simulink model "net_model_2_nodes_ext_switch"  (R2024a)
settings: Solver=VariableStepAuto  StartTime=0.0  StopTime=n_max  RelTol=1e-3
values from neighbouring files (symbols this model uses):
  node_1_0 = [0; 0]    [compute_controller.m]    (also in main.m = [5; 1])
  node_2_0 = [0; 0]    [compute_controller.m]    (also in main.m = [1; 1])
  ss_ctr_fault = ss(ss_fault.A + L2 * ss_fault.C + ss_fault.B * J2, -L2, J2, 0, 1)    [compute_controller.m]
  ss_ctr_nom = ss(ss_nom.A + L1 * ss_nom.C + ss_nom.B * J1, -L1, J1, 0, 1)    [compute_controller.m]
  ss_fault = ss(A, B, C, 0, 1)    [compute_controller.m]
  ss_nom = ss(A, B, C, 0, 1)    [compute_controller.m]
settings Model: Creator=antoniostavarache  LastModifiedBy=antoniostavarache

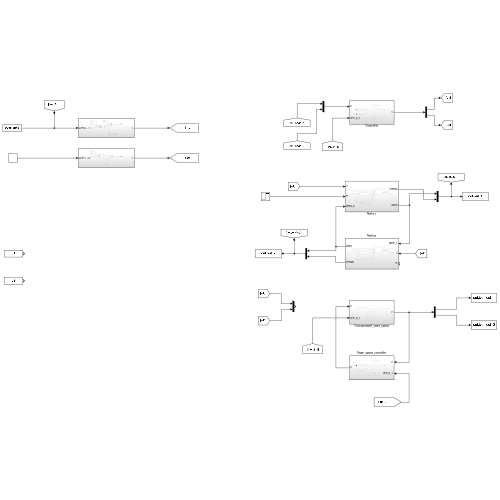
[thumbnail: Simulink's stored preview of the top-level diagram]
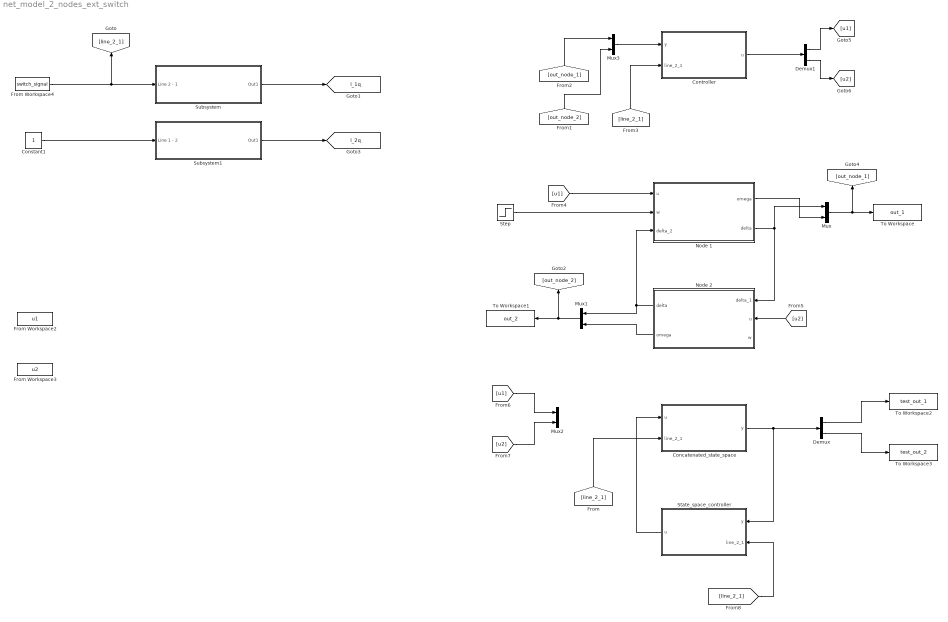
== system net_model_2_nodes_ext_switch ==
  Concatenated_state_space : Subsystem
  Constant1 : Constant
  Controller : Subsystem
  Demux : Demux  Outputs=2
  Demux1 : Demux  Outputs=2
  From Workspace2 : FromWorkspace  VariableName=u1
  From Workspace3 : FromWorkspace  VariableName=u2
  From Workspace4 : FromWorkspace  VariableName=switch_signal  SampleTime=1
  Mux{,1..3} (4 alike) : Mux  Inputs=2
  Node 1 : Subsystem
  Node 2 : Subsystem
  State_space_controller : Subsystem
  Step : Step  Time=250  SampleTime=0
  Subsystem : Subsystem
  Subsystem1 : Subsystem
  To Workspace : ToWorkspace  VariableName=out_1  SaveFormat=Timeseries  SampleTime=-1
  To Workspace1 : ToWorkspace  VariableName=out_2  SaveFormat=Timeseries  SampleTime=-1
  To Workspace2 : ToWorkspace  VariableName=test_out_1  SaveFormat=Timeseries  SampleTime=-1
  To Workspace3 : ToWorkspace  VariableName=test_out_2  SaveFormat=Timeseries  SampleTime=-1
  tag scope: l_1q=global, l_2q=global
  wires:
  Node 1/2(delta) -> Node 2/1(delta_1), Mux/1
  Node 2/1(delta) -> Mux1/1, Node 1/3(delta_2)
  Mux/1 -> To Workspace/1, [out_node_1]
  Mux1/1 -> To Workspace1/1, [out_node_2]
  Node 2/2(omega) -> Mux1/2
  Demux/1 -> To Workspace2/1
  Demux/2 -> To Workspace3/1
  Node 1/1(omega) -> Mux/2
  Subsystem/1(Out1) -> [l_1q]
  Constant1/1 -> Subsystem1/1(Line 1 - 2)
  Subsystem1/1(Out1) -> [l_2q]
  Concatenated_state_space/1(y) -> State_space_controller/1(y), Demux/1
  From Workspace4/1 -> Subsystem/1(Line 2 - 1), [line_2_1]
  [out_node_1] -> Mux3/1
  [out_node_2] -> Mux3/2
  Mux3/1 -> Controller/1(y)
  [line_2_1] -> Controller/2(line_2_1)
  Demux1/1 -> [u1]
  Demux1/2 -> [u2]
  [u1] -> Node 1/1(u)
  [u2] -> Node 2/2(u)
  [line_2_1] -> Concatenated_state_space/2(line_2_1)
  Controller/1(u) -> Demux1/1
  [u1] -> Mux2/1
  [u2] -> Mux2/2
  [line_2_1] -> State_space_controller/2(line_2_1)
  State_space_controller/1(u) -> Concatenated_state_space/1(u)
  Step/1 -> Node 1/2(w)

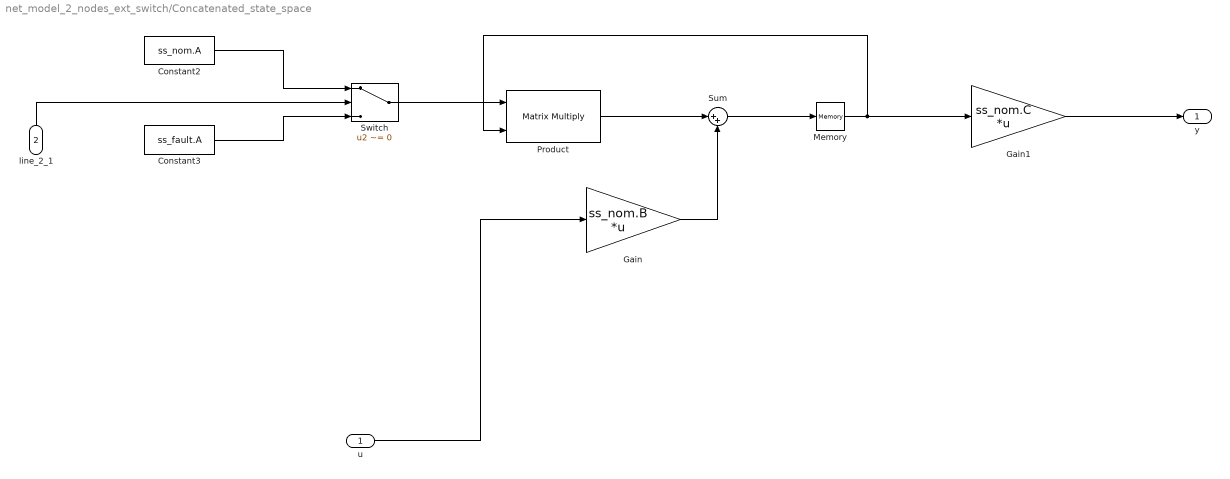
== system net_model_2_nodes_ext_switch/Concatenated_state_space ==
  u : Inport
  line_2_1 : Inport  Port=2
  Constant2 : Constant  Value=ss_nom.A
  Constant3 : Constant  Value=ss_fault.A
  Gain : Gain  Gain=ss_nom.B  Multiplication=Matrix(K*u) (u vector)
  Gain1 : Gain  Gain=ss_nom.C  Multiplication=Matrix(K*u) (u vector)
  Memory : Memory  InitialCondition=[node_1_0; node_2_0]
  Product : Product  Multiplication=Matrix(*)
  Sum : Sum  Inputs=|++
  Switch : Switch  Criteria=u2 ~= 0  SaturateOnIntegerOverflow=off  InputSameDT=off
  y : Outport
  wires:
  Constant3/1 -> Switch/3
  Switch/1 -> Product/1
  Product/1 -> Sum/1
  Memory/1 -> Gain1/1, Product/2
  Gain1/1 -> y/1
  u/1 -> Gain/1
  Sum/1 -> Memory/1
  Gain/1 -> Sum/2
  line_2_1/1 -> Switch/2
  Constant2/1 -> Switch/1

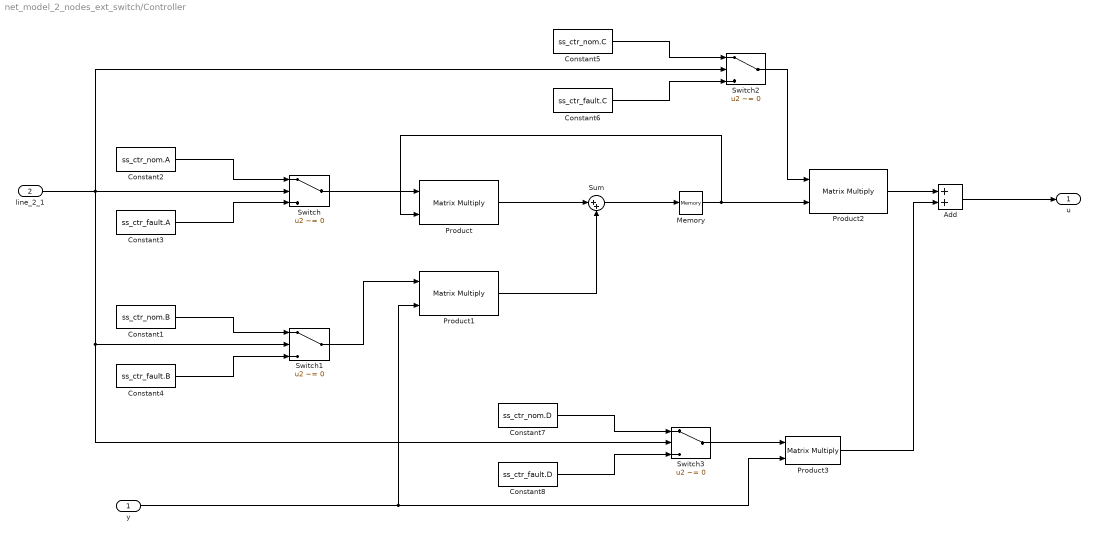
== system net_model_2_nodes_ext_switch/Controller ==
  y : Inport
  line_2_1 : Inport  Port=2
  Add : Sum
  Constant1 : Constant  Value=ss_ctr_nom.B
  Constant2 : Constant  Value=ss_ctr_nom.A
  Constant3 : Constant  Value=ss_ctr_fault.A
  Constant4 : Constant  Value=ss_ctr_fault.B
  Constant5 : Constant  Value=ss_ctr_nom.C
  Constant6 : Constant  Value=ss_ctr_fault.C
  Constant7 : Constant  Value=ss_ctr_nom.D
  Constant8 : Constant  Value=ss_ctr_fault.D
  Memory : Memory  InitialCondition=zeros(4, 1)
  Product{,1..3} (4 alike) : Product  Multiplication=Matrix(*)
  Sum : Sum  Inputs=|++
  Switch{,1..3} (4 alike) : Switch  Criteria=u2 ~= 0  SaturateOnIntegerOverflow=off  InputSameDT=off
  u : Outport
  wires:
  Constant3/1 -> Switch/3
  Switch/1 -> Product/1
  Product/1 -> Sum/1
  Memory/1 -> Product2/2, Product/2
  y/1 -> Product1/2, Product3/2
  Sum/1 -> Memory/1
  Product1/1 -> Sum/2
  line_2_1/1 -> Switch2/2, Switch3/2, Switch1/2, Switch/2
  Constant2/1 -> Switch/1
  Constant4/1 -> Switch1/3
  Constant1/1 -> Switch1/1
  Switch1/1 -> Product1/1
  Constant6/1 -> Switch2/3
  Constant5/1 -> Switch2/1
  Switch2/1 -> Product2/1
  Constant8/1 -> Switch3/3
  Constant7/1 -> Switch3/1
  Product2/1 -> Add/1
  Add/1 -> u/1
  Switch3/1 -> Product3/1
  Product3/1 -> Add/2

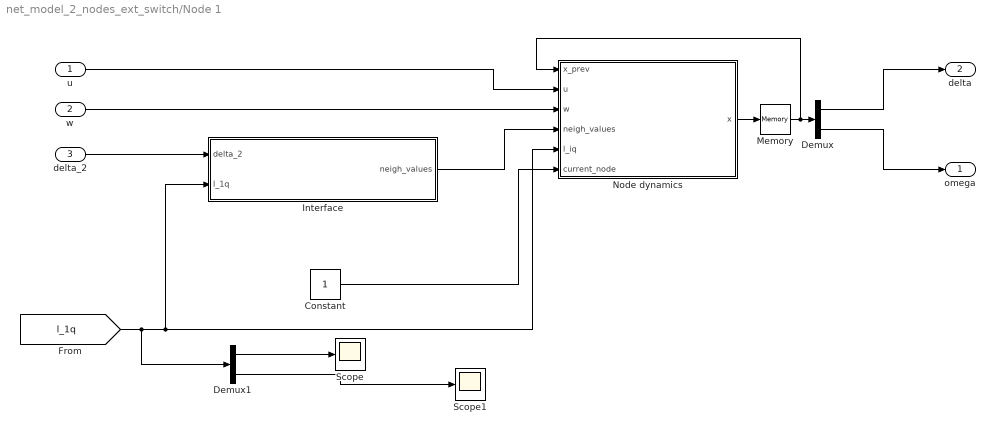
== system net_model_2_nodes_ext_switch/Node 1 ==
  u : Inport
  w : Inport  Port=2
  delta_2 : Inport  Port=3
  Constant : Constant
  Demux : Demux  Outputs=2
  Demux1 : Demux  Outputs=2
  Interface : MATLAB Function  TreatAsAtomicUnit=on
  Memory : Memory  InitialCondition=node_1_0
  Node dynamics : MATLAB Function  TreatAsAtomicUnit=on
  Scope : Scope
  Scope1 : Scope
  omega : Outport
  delta : Outport  Port=2
  wires:
  Node dynamics/1(x) -> Memory/1
  Interface/1(neigh_values) -> Node dynamics/4(neigh_values)
  u/1 -> Node dynamics/2(u)
  w/1 -> Node dynamics/3(w)
  Demux/1 -> delta/1
  Demux/2 -> omega/1
  Memory/1 -> Node dynamics/1(x_prev), Demux/1
  delta_2/1 -> Interface/1(delta_2)
  [l_1q] -> Demux1/1, Node dynamics/5(l_iq), Interface/2(l_1q)
  Constant/1 -> Node dynamics/6(current_node)
  Demux1/1 -> Scope/1
  Demux1/2 -> Scope1/1

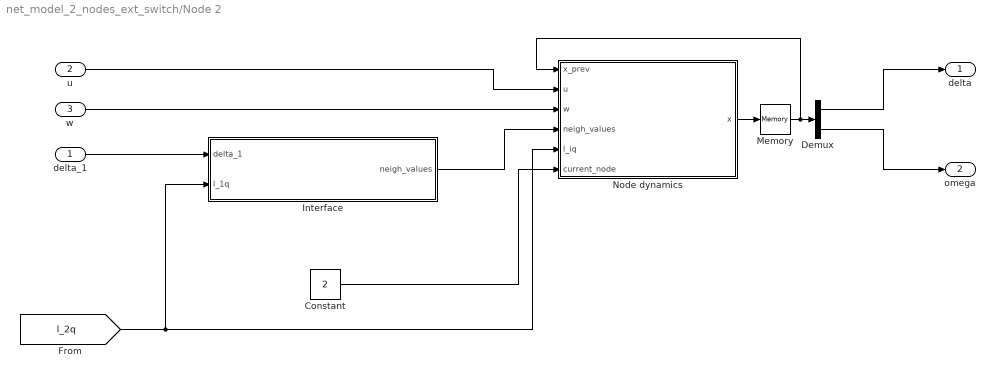
== system net_model_2_nodes_ext_switch/Node 2 ==
  delta_1 : Inport
  u : Inport  Port=2
  w : Inport  Port=3
  Constant : Constant  Value=2
  Demux : Demux  Outputs=2
  Interface : MATLAB Function  TreatAsAtomicUnit=on
  Memory : Memory  InitialCondition=node_2_0
  Node dynamics : MATLAB Function  TreatAsAtomicUnit=on
  delta : Outport
  omega : Outport  Port=2
  wires:
  Node dynamics/1(x) -> Memory/1
  Interface/1(neigh_values) -> Node dynamics/4(neigh_values)
  u/1 -> Node dynamics/2(u)
  w/1 -> Node dynamics/3(w)
  Demux/1 -> delta/1
  Demux/2 -> omega/1
  Memory/1 -> Node dynamics/1(x_prev), Demux/1
  delta_1/1 -> Interface/1(delta_1)
  [l_2q] -> Node dynamics/5(l_iq), Interface/2(l_1q)
  Constant/1 -> Node dynamics/6(current_node)

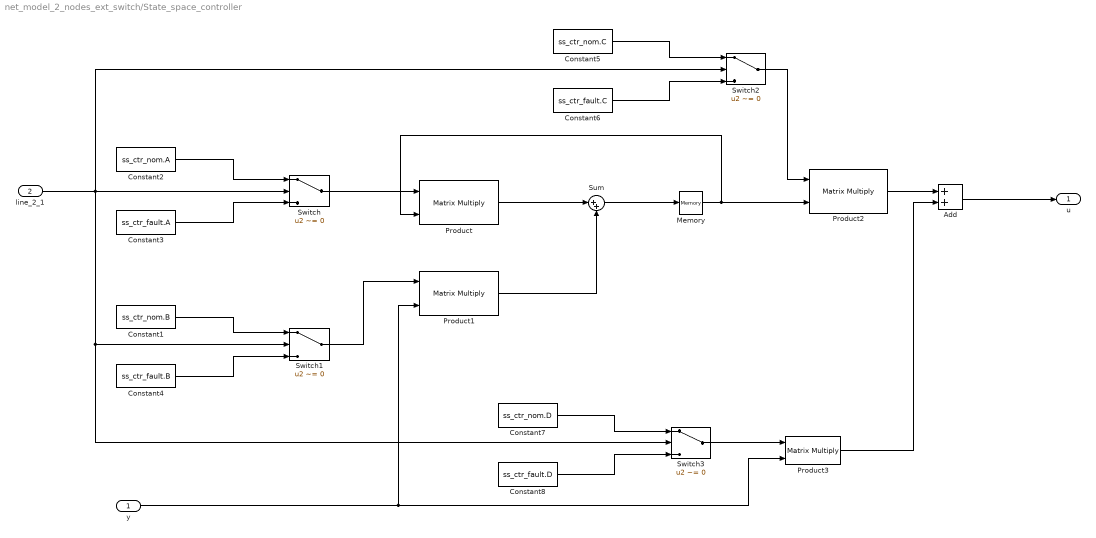
== system net_model_2_nodes_ext_switch/State_space_controller ==
  y : Inport
  line_2_1 : Inport  Port=2
  Add : Sum
  Constant1 : Constant  Value=ss_ctr_nom.B
  Constant2 : Constant  Value=ss_ctr_nom.A
  Constant3 : Constant  Value=ss_ctr_fault.A
  Constant4 : Constant  Value=ss_ctr_fault.B
  Constant5 : Constant  Value=ss_ctr_nom.C
  Constant6 : Constant  Value=ss_ctr_fault.C
  Constant7 : Constant  Value=ss_ctr_nom.D
  Constant8 : Constant  Value=ss_ctr_fault.D
  Memory : Memory  InitialCondition=zeros(4, 1)
  Product{,1..3} (4 alike) : Product  Multiplication=Matrix(*)
  Sum : Sum  Inputs=|++
  Switch{,1..3} (4 alike) : Switch  Criteria=u2 ~= 0  SaturateOnIntegerOverflow=off  InputSameDT=off
  u : Outport
  wires:
  Constant3/1 -> Switch/3
  Switch/1 -> Product/1
  Product/1 -> Sum/1
  Memory/1 -> Product2/2, Product/2
  y/1 -> Product1/2, Product3/2
  Sum/1 -> Memory/1
  Product1/1 -> Sum/2
  line_2_1/1 -> Switch2/2, Switch3/2, Switch1/2, Switch/2
  Constant2/1 -> Switch/1
  Constant4/1 -> Switch1/3
  Constant1/1 -> Switch1/1
  Switch1/1 -> Product1/1
  Constant6/1 -> Switch2/3
  Constant5/1 -> Switch2/1
  Switch2/1 -> Product2/1
  Constant8/1 -> Switch3/3
  Constant7/1 -> Switch3/1
  Product2/1 -> Add/1
  Add/1 -> u/1
  Switch3/1 -> Product3/1
  Product3/1 -> Add/2

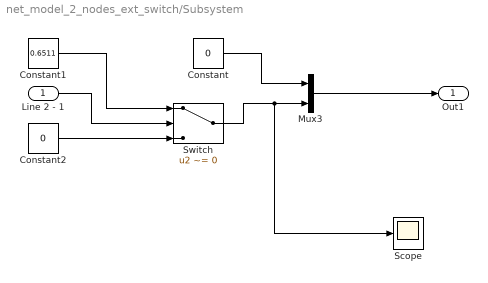
== system net_model_2_nodes_ext_switch/Subsystem ==
  Line 2 - 1 : Inport
  Constant : Constant  Value=0
  Constant1 : Constant  Value=0.6511
  Constant2 : Constant  Value=0
  Mux3 : Mux  Inputs=2
  Scope : Scope
  Switch : Switch  Criteria=u2 ~= 0  SaturateOnIntegerOverflow=off  InputSameDT=off
  Out1 : Outport
  wires:
  Mux3/1 -> Out1/1
  Line 2 - 1/1 -> Switch/2
  Constant/1 -> Mux3/1
  Switch/1 -> Scope/1, Mux3/2
  Constant2/1 -> Switch/3
  Constant1/1 -> Switch/1

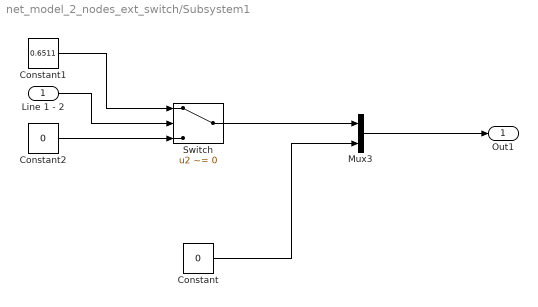
== system net_model_2_nodes_ext_switch/Subsystem1 ==
  Line 1 - 2 : Inport
  Constant : Constant  Value=0
  Constant1 : Constant  Value=0.6511
  Constant2 : Constant  Value=0
  Mux3 : Mux  Inputs=2
  Switch : Switch  Criteria=u2 ~= 0  SaturateOnIntegerOverflow=off  InputSameDT=off
  Out1 : Outport
  wires:
  Mux3/1 -> Out1/1
  Line 1 - 2/1 -> Switch/2
  Switch/1 -> Mux3/1
  Constant2/1 -> Switch/3
  Constant1/1 -> Switch/1
  Constant/1 -> Mux3/2

== matlab function net_model_2_nodes_ext_switch/Node 1/Interface ==
  data: delta_2 input; neigh_values output; l_1q input
function neigh_values = fcn(delta_2, l_1q)

    neigh_values = l_1q(2) * delta_2;

end

== matlab function net_model_2_nodes_ext_switch/Node 1/Node dynamics ==
  data: x_prev input; u input; x output; w input; neigh_values input; l_iq input; current_node input
function x = fcn(x_prev, u, w, neigh_values, l_iq, current_node)
    
    % current_node = 1;

%%

    hi = [0.3244
        1.5886];

    di = [0.5650;
        0.7844];

    dt = 0.2;
%%

    a21 = -hi(current_node) * dt * sum(l_iq);
    a22 = 1 - hi(current_node) * di(current_node) * dt;

    A = [1, dt;
        a21, a22];

    x = A * x_prev + [0 1]' * (u + w + hi(current_node) * dt * neigh_values);
    
end

== matlab function net_model_2_nodes_ext_switch/Node 2/Interface ==
  data: delta_1 input; neigh_values output; l_1q input
function neigh_values = fcn(delta_1, l_1q)

    neigh_values = l_1q(1) * delta_1;

end

== matlab function net_model_2_nodes_ext_switch/Node 2/Node dynamics ==
  data: x_prev input; u input; x output; w input; neigh_values input; l_iq input; current_node input
function x = fcn(x_prev, u, w, neigh_values, l_iq, current_node)
    
    % current_node = 1;

%%

    hi = [0.3244
        1.5886];

    di = [0.5650;
        0.7844];

    dt = 0.2;
%%

    a21 = -hi(current_node) * dt * sum(l_iq);
    a22 = 1 - hi(current_node) * di(current_node) * dt;

    A = [1, dt;
        a21, a22];

    x = A * x_prev + [0 1]' * (u + w + hi(current_node) * dt * neigh_values);
    
end
